simulink model "Test_ex_mp_switch_block_noncontiguous_indices1"  (R2015a)
settings: Solver=FixedStepDiscrete  StartTime=0.0  StopTime=10.0  FixedStep=0.1  RelTol=1e-3
settings Model: Creator=The MathWorks Inc.  LastModifiedBy=think0404
settings OptimizationCC: ExpressionDepthLimit=2147483647
settings DebuggingCC: UnderspecifiedInitializationDetection=Classic  MergeDetectMultiDrivingBlocksExec=none  SolverPrmCheckMsg=warning  FcnCallInpInsideContextMsg=UseLocalSettings  StateNameClashWarn=warning
settings GRTTargetCC: CombineOutputUpdateFcns=off  GRTInterface=on

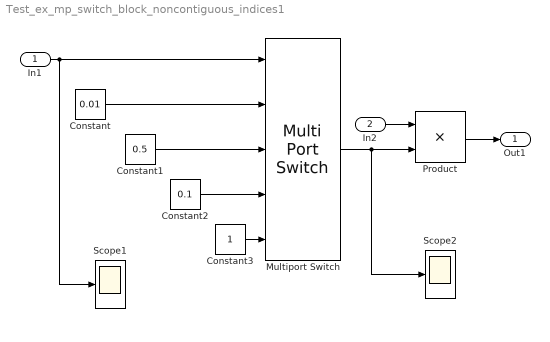
== system Test_ex_mp_switch_block_noncontiguous_indices1 ==
  In1 : Inport
  In2 : Inport  Port=2
  Constant : Constant  Value=0.01
  Constant1 : Constant  Value=0.5
  Constant2 : Constant  Value=0.1
  Constant3 : Constant
  Multiport Switch : MultiPortSwitch  DataPortOrder=Specify indices  DataPortIndices={[3,5],0,18}  DataPortForDefault=Additional data port
  Product : Product  RndMeth=Zero
  Scope1 : Scope
      settings: TimeRange=0.1  YMin=-2  SaveName=VI2  Decimation=10
  Scope2 : Scope
      settings: TimeRange=0.1  YMin=-2  SaveName=VI  Decimation=10
  Out1 : Outport
  wires:
  In1/1 -> Scope1/1, Multiport Switch/1
  Multiport Switch/1 -> Scope2/1, Product/2
  In2/1 -> Product/1
  Constant/1 -> Multiport Switch/2
  Constant1/1 -> Multiport Switch/3
  Constant2/1 -> Multiport Switch/4
  Product/1 -> Out1/1
  Constant3/1 -> Multiport Switch/5
